simulink model "muscleLegs_task1"  (R2025b)
settings: Solver=ode23t  StartTime=0.0  StopTime=t_end  MaxStep=1e-3  RelTol=1e-4
values from neighbouring files (symbols this model uses):
  c = 0.05    [setup_muscleLegs_nm.m]
  CtrlPar = [tau_H_st; phi_K_tgt_st; P_K_st; D_K_st ... (first row only)    [setup_muscleLegs_ctrl.m]
  eref_se = 0.04    [setup_muscleLegs_nm.m]
  FmaxBFSH = 350    [setup_muscleLegs_nm.m]
  FmaxGLU = 4000    [setup_muscleLegs_nm.m]
  FmaxHFL = 2000    [setup_muscleLegs_nm.m]
  FmaxVAS = 5000    [setup_muscleLegs_nm.m]
  g = 9.81    [setup_muscleLegs_model.m]
  init_stim = 0.01    [setup_muscleLegs_nm.m]
  K = 5    [setup_muscleLegs_nm.m]
  l_shank = l_leg/2    (= 0.49)    [setup_muscleLegs_model.m]
  l_thigh = l_leg/2    (= 0.49)    [setup_muscleLegs_model.m]
  loptBFSH = 0.12    [setup_muscleLegs_nm.m]
  loptGLU = 0.11    [setup_muscleLegs_nm.m]
  loptHFL = 0.11    [setup_muscleLegs_nm.m]
  loptVAS = 0.08    [setup_muscleLegs_nm.m]
  lslackBFSH = 0.10    (= 0.1)    [setup_muscleLegs_nm.m]
  lslackGLU = 0.13    [setup_muscleLegs_nm.m]
  lslackHFL = 0.10    (= 0.1)    [setup_muscleLegs_nm.m]
  lslackVAS = 0.23    [setup_muscleLegs_nm.m]
  m_body = m_total - 2*m_foot    (= 78)    [setup_muscleLegs_model.m]
  m_shank = 4    [setup_muscleLegs_model.m]
  m_thigh = 8    [setup_muscleLegs_model.m]
  N = 12    [cmaes_task1_2_set1.mat]    (also in cmaes_task1_2_set2.mat; cmaes_task2_2_set1.mat = 17; cmaes_task2_2_set2.mat = 17; cmaes_task3_crouch.mat = 17)
  phirefBFSH = 160*pi/180    (= 2.79252680319)    [setup_muscleLegs_nm.m]
  phirefGLU = 60*pi/180    (= 1.0471975512)    [setup_muscleLegs_nm.m]
  phirefHFL = 20*pi/180    (= 0.349065850399)    [setup_muscleLegs_nm.m]
  phirefVAS = 60*pi/180    (= 1.0471975512)    [setup_muscleLegs_nm.m]
  plane_height = 0.1    [setup_muscleLegs_model.m]
  plane_x = 100    [setup_muscleLegs_model.m]
  plane_z = 1    [setup_muscleLegs_model.m]
  r_foot = 0.01    [setup_muscleLegs_model.m]
  rBFSH = 0.04    [setup_muscleLegs_nm.m]
  rGLU = 0.08    [setup_muscleLegs_nm.m]
  rHFL = 0.08    [setup_muscleLegs_nm.m]
  rhoBFSH = 0.7    [setup_muscleLegs_nm.m]
  rhoGLU = 0.5    [setup_muscleLegs_nm.m]
  rhoHFL = 0.5    [setup_muscleLegs_nm.m]
  rhoVAS = 0.6    [setup_muscleLegs_nm.m]
  rVAS = 0.05    [setup_muscleLegs_nm.m]
  tau_act = 0.01    [setup_muscleLegs_nm.m]
  tau_deact = 0.04    [setup_muscleLegs_nm.m]
  vi_Ctrl_st = 1:4    [setup_muscleLegs_ctrl.m]
  vi_Ctrl_sw = 5:12    [setup_muscleLegs_ctrl.m]
  vmaxBFSH = 12    [setup_muscleLegs_nm.m]
  vmaxGLU = 12    [setup_muscleLegs_nm.m]
  vmaxHFL = 12    [setup_muscleLegs_nm.m]
  vmaxVAS = 12    [setup_muscleLegs_nm.m]
  w = 0.56    [setup_muscleLegs_nm.m]
  w_pe = w    (= 0.56)    [setup_muscleLegs_nm.m]
undefined symbols (not defined in the file or in its folder): l1, X, Y, Z
libraries: sm_lib x30, nesl_utility x17, simulink x1
(part 2 of 4)

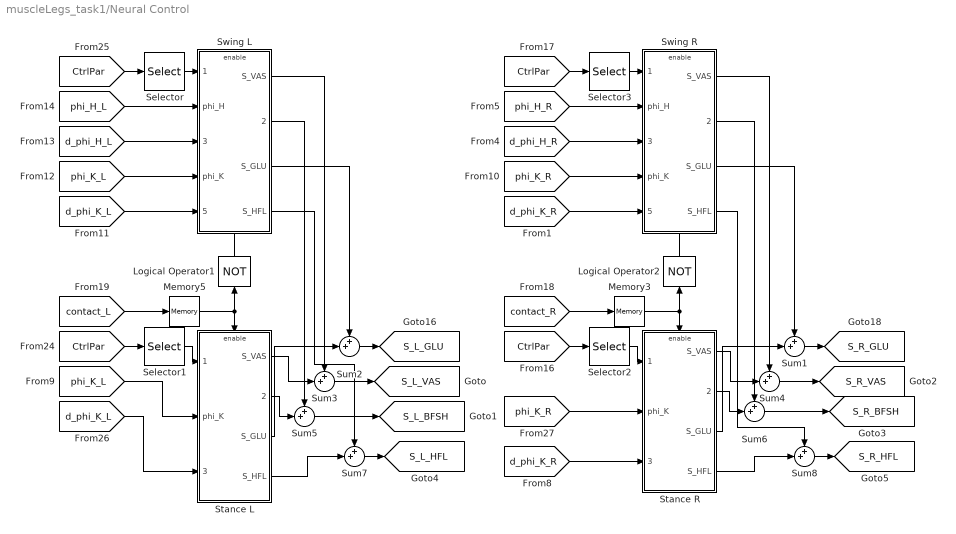
== system muscleLegs_task1/Neural Control ==
  Logical Operator1 : Logic  Operator=NOT  AllPortsSameDT=off  OutDataTypeStr=boolean
  Logical Operator2 : Logic  Operator=NOT  AllPortsSameDT=off  OutDataTypeStr=boolean
  Memory3 : Memory
  Memory5 : Memory  InitialCondition=1
  Selector : Selector  InputPortWidth=length(CtrlPar)  IndexOptions=Index vector (dialog)  Indices=vi_Ctrl_sw  OutputSizes=1
  Selector1 : Selector  InputPortWidth=length(CtrlPar)  IndexOptions=Index vector (dialog)  Indices=vi_Ctrl_st  OutputSizes=1
  Selector2 : Selector  InputPortWidth=length(CtrlPar)  IndexOptions=Index vector (dialog)  Indices=vi_Ctrl_st  OutputSizes=1
  Selector3 : Selector  InputPortWidth=length(CtrlPar)  IndexOptions=Index vector (dialog)  Indices=vi_Ctrl_sw  OutputSizes=1
  Stance L : Subsystem
  Stance R : Subsystem
  Sum{1..8} (8 alike) : Sum  Inputs=++|
  Swing L : Subsystem
  Swing R : Subsystem
  tag scope: S_L_BFSH=global, S_L_GLU=global, S_L_HFL=global, S_L_VAS=global, S_R_BFSH=global, S_R_GLU=global, S_R_HFL=global, S_R_VAS=global
  wires:
  [contact_R] -> Memory3/1
  [phi_K_R] -> Swing R/4(phi_K)
  Sum2/1 -> [S_L_GLU]
  Logical Operator1/1 -> Swing L/Enable
  Memory5/1 -> Logical Operator1/1, Stance L/Enable
  Selector1/1 -> Stance L/1(CtrlPar)
  [CtrlPar] -> Selector2/1
  Memory3/1 -> Stance R/Enable, Logical Operator2/1
  [phi_H_L] -> Swing L/2(phi_H)
  [d_phi_K_L] -> Stance L/3(d_phi_K)
  Logical Operator2/1 -> Swing R/Enable
  [d_phi_K_R] -> Stance R/3(d_phi_K)
  [d_phi_H_L] -> Swing L/3(d_phi_H)
  Sum1/1 -> [S_R_GLU]
  [d_phi_K_L] -> Swing L/5(d_phi_K)
  [d_phi_H_R] -> Swing R/3(d_phi_H)
  [d_phi_K_R] -> Swing R/5(d_phi_K)
  [phi_H_R] -> Swing R/2(phi_H)
  [CtrlPar] -> Selector/1
  [CtrlPar] -> Selector1/1
  Selector3/1 -> Swing R/1(CtrlPar)
  [phi_K_R] -> Stance R/2(phi_K)
  Selector/1 -> Swing L/1(CtrlPar)
  Selector2/1 -> Stance R/1(CtrlPar)
  [CtrlPar] -> Selector3/1
  [phi_K_L] -> Stance L/2(phi_K)
  [phi_K_L] -> Swing L/4(phi_K)
  [contact_L] -> Memory5/1
  Swing L/1(S_VAS) -> Sum3/1
  Swing L/2(S_BFSH) -> Sum5/1
  Sum3/1 -> [S_L_VAS]
  Stance L/1(S_VAS) -> Sum3/2
  Stance L/2(S_BFSH) -> Sum5/2
  Sum5/1 -> [S_L_BFSH]
  Stance R/2(S_BFSH) -> Sum6/2
  Stance R/1(S_VAS) -> Sum4/2
  Sum4/1 -> [S_R_VAS]
  Sum6/1 -> [S_R_BFSH]
  Swing R/2(S_BFSH) -> Sum6/1
  Swing R/1(S_VAS) -> Sum4/1
  Swing L/3(S_GLU) -> Sum2/1
  Stance L/3(S_GLU) -> Sum2/2
  Sum7/1 -> [S_L_HFL]
  Swing L/4(S_HFL) -> Sum7/1
  Stance L/4(S_HFL) -> Sum7/2
  Swing R/3(S_GLU) -> Sum1/1
  Stance R/3(S_GLU) -> Sum1/2
  Sum8/1 -> [S_R_HFL]
  Swing R/4(S_HFL) -> Sum8/1
  Stance R/4(S_HFL) -> Sum8/2

== system muscleLegs_task1/Muscle Dynamics/ECC ==
  S : Inport
  Constant : Constant  Value=tau_act
  Constant1 : Constant  Value=tau_deact
  Divide : Product  Inputs=*/
  Integrator : Integrator  InitialCondition=init_stim
  Sum : Sum  Inputs=+-|
  Switch : Switch  Criteria=u2 > Threshold  SaturateOnIntegerOverflow=off  InputSameDT=off
  Out1 : Outport
  A : Outport  Port=2  VectorParamsAs1DForOutWhenUnconnected=off
  wires:
  S/1 -> Sum/1
  Integrator/1 -> A/1, Sum/2  "A"
  Divide/1 -> Integrator/1  "dA"
  Sum/1 -> Divide/1, Switch/2
  Switch/1 -> Divide/2
  Constant/1 -> Switch/1
  Constant1/1 -> Switch/3

== system muscleLegs_task1/Muscle Dynamics/ECC1 ==
  S : Inport
  Constant : Constant  Value=tau_act
  Constant1 : Constant  Value=tau_deact
  Divide : Product  Inputs=*/
  Integrator : Integrator  InitialCondition=init_stim
  Sum : Sum  Inputs=+-|
  Switch : Switch  Criteria=u2 > Threshold  SaturateOnIntegerOverflow=off  InputSameDT=off
  A : Outport  VectorParamsAs1DForOutWhenUnconnected=off
  wires:
  S/1 -> Sum/1
  Integrator/1 -> A/1, Sum/2  "A"
  Divide/1 -> Integrator/1  "dA"
  Sum/1 -> Divide/1, Switch/2
  Switch/1 -> Divide/2
  Constant/1 -> Switch/1
  Constant1/1 -> Switch/3

== system muscleLegs_task1/Muscle Dynamics/ECC2 ==
  S : Inport
  Constant : Constant  Value=tau_act
  Constant1 : Constant  Value=tau_deact
  Divide : Product  Inputs=*/
  Integrator : Integrator  InitialCondition=init_stim
  Sum : Sum  Inputs=+-|
  Switch : Switch  Criteria=u2 > Threshold  SaturateOnIntegerOverflow=off  InputSameDT=off
  A : Outport  VectorParamsAs1DForOutWhenUnconnected=off
  wires:
  S/1 -> Sum/1
  Integrator/1 -> A/1, Sum/2  "A"
  Divide/1 -> Integrator/1  "dA"
  Sum/1 -> Divide/1, Switch/2
  Switch/1 -> Divide/2
  Constant/1 -> Switch/1
  Constant1/1 -> Switch/3

== system muscleLegs_task1/Muscle Dynamics/ECC3 ==
  S : Inport
  Constant : Constant  Value=tau_act
  Constant1 : Constant  Value=tau_deact
  Divide : Product  Inputs=*/
  Integrator : Integrator  InitialCondition=init_stim
  Sum : Sum  Inputs=+-|
  Switch : Switch  Criteria=u2 > Threshold  SaturateOnIntegerOverflow=off  InputSameDT=off
  A : Outport  VectorParamsAs1DForOutWhenUnconnected=off
  wires:
  S/1 -> Sum/1
  Integrator/1 -> A/1, Sum/2  "A"
  Divide/1 -> Integrator/1  "dA"
  Sum/1 -> Divide/1, Switch/2
  Switch/1 -> Divide/2
  Constant/1 -> Switch/1
  Constant1/1 -> Switch/3

== system muscleLegs_task1/Muscle Dynamics/ECC4 ==
  S : Inport
  Constant : Constant  Value=tau_act
  Constant1 : Constant  Value=tau_deact
  Divide : Product  Inputs=*/
  Integrator : Integrator  InitialCondition=init_stim
  Sum : Sum  Inputs=+-|
  Switch : Switch  Criteria=u2 > Threshold  SaturateOnIntegerOverflow=off  InputSameDT=off
  A : Outport  VectorParamsAs1DForOutWhenUnconnected=off
  wires:
  S/1 -> Sum/1
  Integrator/1 -> A/1, Sum/2  "A"
  Divide/1 -> Integrator/1  "dA"
  Sum/1 -> Divide/1, Switch/2
  Switch/1 -> Divide/2
  Constant/1 -> Switch/1
  Constant1/1 -> Switch/3

== system muscleLegs_task1/Muscle Dynamics/ECC5 ==
  S : Inport
  Constant : Constant  Value=tau_act
  Constant1 : Constant  Value=tau_deact
  Divide : Product  Inputs=*/
  Integrator : Integrator  InitialCondition=init_stim
  Sum : Sum  Inputs=+-|
  Switch : Switch  Criteria=u2 > Threshold  SaturateOnIntegerOverflow=off  InputSameDT=off
  A : Outport  VectorParamsAs1DForOutWhenUnconnected=off
  wires:
  S/1 -> Sum/1
  Integrator/1 -> A/1, Sum/2  "A"
  Divide/1 -> Integrator/1  "dA"
  Sum/1 -> Divide/1, Switch/2
  Switch/1 -> Divide/2
  Constant/1 -> Switch/1
  Constant1/1 -> Switch/3

== system muscleLegs_task1/Muscle Dynamics/ECC6 ==
  S : Inport
  Constant : Constant  Value=tau_act
  Constant1 : Constant  Value=tau_deact
  Divide : Product  Inputs=*/
  Integrator : Integrator  InitialCondition=init_stim
  Sum : Sum  Inputs=+-|
  Switch : Switch  Criteria=u2 > Threshold  SaturateOnIntegerOverflow=off  InputSameDT=off
  A : Outport  VectorParamsAs1DForOutWhenUnconnected=off
  wires:
  S/1 -> Sum/1
  Integrator/1 -> A/1, Sum/2  "A"
  Divide/1 -> Integrator/1  "dA"
  Sum/1 -> Divide/1, Switch/2
  Switch/1 -> Divide/2
  Constant/1 -> Switch/1
  Constant1/1 -> Switch/3

== system muscleLegs_task1/Muscle Dynamics/ECC7 ==
  S : Inport
  Constant : Constant  Value=tau_act
  Constant1 : Constant  Value=tau_deact
  Divide : Product  Inputs=*/
  Integrator : Integrator  InitialCondition=init_stim
  Sum : Sum  Inputs=+-|
  Switch : Switch  Criteria=u2 > Threshold  SaturateOnIntegerOverflow=off  InputSameDT=off
  A : Outport  VectorParamsAs1DForOutWhenUnconnected=off
  wires:
  S/1 -> Sum/1
  Integrator/1 -> A/1, Sum/2  "A"
  Divide/1 -> Integrator/1  "dA"
  Sum/1 -> Divide/1, Switch/2
  Switch/1 -> Divide/2
  Constant/1 -> Switch/1
  Constant1/1 -> Switch/3

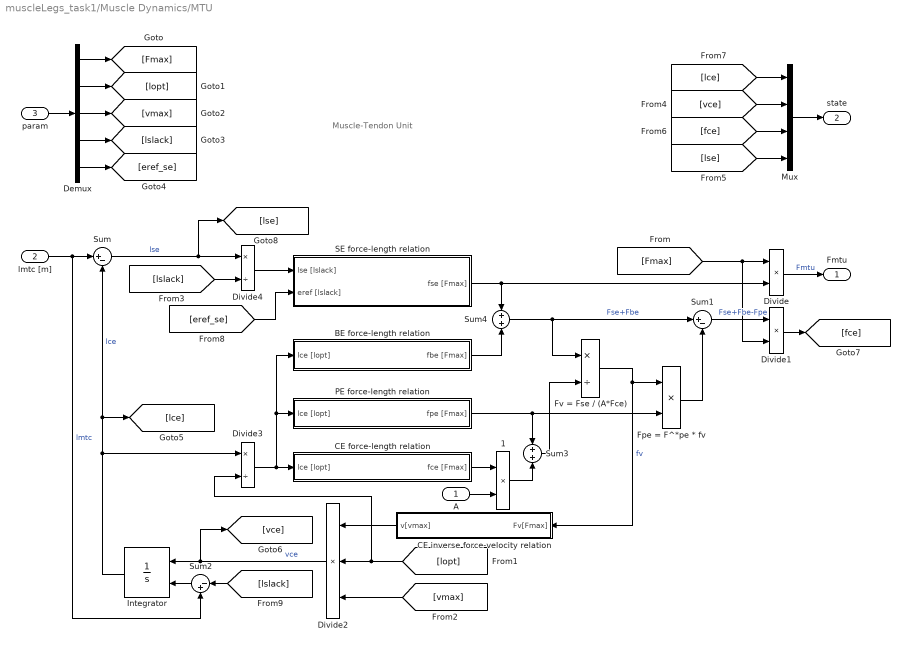
== system muscleLegs_task1/Muscle Dynamics/MTU ==
  note: Muscle-Tendon Unit
  A : Inport
  lmtc [m] : Inport  Port=2
  param : Inport  Port=3
  1 : Product  Inputs=**  InputSameDT=on  SaturateOnIntegerOverflow=on  OutDataTypeStr=Inherit: Same as first input
  BE force-length relation : Subsystem
  CE force-length relation : Subsystem
  CE inverse force-velocity relation : Subsystem
  Demux : Demux  Outputs=5
  Divide : Product
  Divide1 : Product
  Divide2 : Product  Inputs=3
  Divide3 : Product  Inputs=*/
  Divide4 : Product  Inputs=*/
  "Fpe = F^*pe * fv " : Product  InputSameDT=on  SaturateOnIntegerOverflow=on  OutDataTypeStr=Inherit: Same as first input
  Fv = Fse / (A*Fce) : Product  Inputs=*/  InputSameDT=on  SaturateOnIntegerOverflow=on  OutDataTypeStr=Inherit: Same as first input
  Integrator : Integrator  InitialConditionSource=external  LowerSaturationLimit=0.05
  Mux : Mux
  PE force-length relation : Subsystem
  SE force-length relation : Subsystem
  Sum : Sum  Inputs=|+-  InputSameDT=on  SaturateOnIntegerOverflow=on  OutDataTypeStr=Inherit: Same as first input
  Sum1 : Sum  Inputs=|+-  InputSameDT=on  SaturateOnIntegerOverflow=on  OutDataTypeStr=Inherit: Same as first input
  Sum2 : Sum  Inputs=|-+  InputSameDT=on  SaturateOnIntegerOverflow=on  OutDataTypeStr=Inherit: Same as first input
  Sum3 : Sum  InputSameDT=on  SaturateOnIntegerOverflow=on  OutDataTypeStr=Inherit: Same as first input
  Sum4 : Sum  InputSameDT=on  SaturateOnIntegerOverflow=on  OutDataTypeStr=Inherit: Same as first input
  Fmtu : Outport  InitialOutput=0  VectorParamsAs1DForOutWhenUnconnected=off
  state : Outport  Port=2  InitialOutput=0  VectorParamsAs1DForOutWhenUnconnected=off
  wires:
  Integrator/1 -> Divide3/1, [lce], Sum/2  "lce"
  Divide3/1 -> CE force-length relation/1(lce [lopt]), PE force-length relation/1(lce [lopt]), BE force-length relation/1(lce [lopt])
  Fv = Fse / (A*Fce)/1 -> CE inverse force-velocity relation/1(Fv[Fmax]), "Fpe = F^*pe * fv "/1  "fv"
  Divide2/1 -> [vce], Integrator/1  "vce"
  lmtc [m]/1 -> Sum/1, Sum2/2  "lmtc"
  Divide/1 -> Fmtu/1  "Fmtu"
  Divide4/1 -> SE force-length relation/1(lse [lslack])
  SE force-length relation/1(fse [Fmax]) -> Sum4/1, Divide/2
  Sum2/1 -> Integrator/2
  [lslack] -> Sum2/1
  CE force-length relation/1(fce [Fmax]) -> 1/1
  PE force-length relation/1(fpe [Fmax]) -> "Fpe = F^*pe * fv "/2, Sum3/1
  1/1 -> Sum3/2
  BE force-length relation/1(fbe [Fmax]) -> Sum4/2
  Sum3/1 -> Fv = Fse / (A*Fce)/2
  CE inverse force-velocity relation/1(v[vmax]) -> Divide2/1
  A/1 -> 1/2
  Sum4/1 -> Sum1/1, Fv = Fse / (A*Fce)/1  "Fse+Fbe"
  "Fpe = F^*pe * fv "/1 -> Sum1/2
  Sum1/1 -> Divide1/1  "Fse+Fbe-Fpe"
  Divide1/1 -> [fce]
  Sum/1 -> [lse], Divide4/1  "lse"
  [lopt] -> Divide2/2, Divide3/2
  [vmax] -> Divide2/3
  [lslack] -> Divide4/2
  param/1 -> Demux/1
  Demux/1 -> [Fmax]
  Demux/2 -> [lopt]
  Demux/4 -> [lslack]
  Demux/3 -> [vmax]
  Demux/5 -> [eref_se]
  [Fmax] -> Divide1/2, Divide/1
  Mux/1 -> state/1
  [lce] -> Mux/1
  [vce] -> Mux/2
  [fce] -> Mux/3
  [lse] -> Mux/4
  [eref_se] -> SE force-length relation/2(eref [lslack])

== system muscleLegs_task1/Muscle Dynamics/MTU Link ==
  note: check sign:
      | ++: larger phi -> longer mtu
      | +-: larger phi -> shorter mtu
  note: Muscle Attachment
  phi [rad] : Inport
  param : Inport  Port=2
  Demux : Demux  Outputs=5
  Product : Product  Inputs=3  RndMeth=Zero
  Sum1 : Sum  Inputs=|++
  Sum2 : Sum  Inputs=|+-
  Sum5 : Sum  Inputs=|++
  lmtu [m] : Outport  VectorParamsAs1DForOutWhenUnconnected=off
  lever [m] : Outport  Port=2  VectorParamsAs1DForOutWhenUnconnected=off
  wires:
  Sum1/1 -> Sum5/1
  Sum5/1 -> lmtu [m]/1
  phi [rad]/1 -> Sum2/1
  Demux/3 -> Sum2/2  "phiref"
  Sum2/1 -> Product/1
  Demux/4 -> lever [m]/1, Product/2  "r"
  Product/1 -> Sum5/2
  Demux/1 -> Sum1/1  "lopt"
  Demux/2 -> Sum1/2  "lslack"
  Demux/5 -> Product/3  "rho"
  param/1 -> Demux/1

== system muscleLegs_task1/Muscle Dynamics/MTU Link1 ==
  note: check sign:
      | ++: larger phi -> longer mtu
      | +-: larger phi -> shorter mtu
  note: Muscle Attachment
  phi [rad] : Inport
  param : Inport  Port=2
  Demux : Demux  Outputs=5
  Product : Product  Inputs=3  RndMeth=Zero
  Sum1 : Sum  Inputs=|++
  Sum2 : Sum  Inputs=|+-
  Sum5 : Sum  Inputs=|+-
  lmtu [m] : Outport  VectorParamsAs1DForOutWhenUnconnected=off
  lever [m] : Outport  Port=2  VectorParamsAs1DForOutWhenUnconnected=off
  wires:
  Sum1/1 -> Sum5/1
  Sum5/1 -> lmtu [m]/1
  phi [rad]/1 -> Sum2/1
  Demux/3 -> Sum2/2  "phiref"
  Sum2/1 -> Product/1
  Demux/4 -> lever [m]/1, Product/2  "r"
  Product/1 -> Sum5/2
  Demux/1 -> Sum1/1  "lopt"
  Demux/2 -> Sum1/2  "lslack"
  Demux/5 -> Product/3  "rho"
  param/1 -> Demux/1

== system muscleLegs_task1/Muscle Dynamics/MTU Link2 ==
  note: check sign:
      | ++: larger phi -> longer mtu
      | +-: larger phi -> shorter mtu
  note: Muscle Attachment
  phi [rad] : Inport
  param : Inport  Port=2
  Demux : Demux  Outputs=5
  Product : Product  Inputs=3  RndMeth=Zero
  Sum1 : Sum  Inputs=|++
  Sum2 : Sum  Inputs=|+-
  Sum5 : Sum  Inputs=|++
  lmtu [m] : Outport  VectorParamsAs1DForOutWhenUnconnected=off
  lever [m] : Outport  Port=2  VectorParamsAs1DForOutWhenUnconnected=off
  wires:
  Sum1/1 -> Sum5/1
  Sum5/1 -> lmtu [m]/1
  phi [rad]/1 -> Sum2/1
  Demux/3 -> Sum2/2  "phiref"
  Sum2/1 -> Product/1
  Demux/4 -> lever [m]/1, Product/2  "r"
  Product/1 -> Sum5/2
  Demux/1 -> Sum1/1  "lopt"
  Demux/2 -> Sum1/2  "lslack"
  Demux/5 -> Product/3  "rho"
  param/1 -> Demux/1

== system muscleLegs_task1/Muscle Dynamics/MTU Link3 ==
  note: check sign:
      | ++: larger phi -> longer mtu
      | +-: larger phi -> shorter mtu
  note: Muscle Attachment
  phi [rad] : Inport
  param : Inport  Port=2
  Demux : Demux  Outputs=5
  Product : Product  Inputs=3  RndMeth=Zero
  Sum1 : Sum  Inputs=|++
  Sum2 : Sum  Inputs=|+-
  Sum5 : Sum  Inputs=|+-
  lmtu [m] : Outport  VectorParamsAs1DForOutWhenUnconnected=off
  lever [m] : Outport  Port=2  VectorParamsAs1DForOutWhenUnconnected=off
  wires:
  Sum1/1 -> Sum5/1
  Sum5/1 -> lmtu [m]/1
  phi [rad]/1 -> Sum2/1
  Demux/3 -> Sum2/2  "phiref"
  Sum2/1 -> Product/1
  Demux/4 -> lever [m]/1, Product/2  "r"
  Product/1 -> Sum5/2
  Demux/1 -> Sum1/1  "lopt"
  Demux/2 -> Sum1/2  "lslack"
  Demux/5 -> Product/3  "rho"
  param/1 -> Demux/1

== system muscleLegs_task1/Muscle Dynamics/MTU Link4 ==
  note: check sign:
      | ++: larger phi -> longer mtu
      | +-: larger phi -> shorter mtu
  note: Muscle Attachment
  phi [rad] : Inport
  param : Inport  Port=2
  Demux : Demux  Outputs=5
  Product : Product  Inputs=3  RndMeth=Zero
  Sum1 : Sum  Inputs=|++
  Sum2 : Sum  Inputs=|+-
  Sum5 : Sum  Inputs=|++
  lmtu [m] : Outport  VectorParamsAs1DForOutWhenUnconnected=off
  lever [m] : Outport  Port=2  VectorParamsAs1DForOutWhenUnconnected=off
  wires:
  Sum1/1 -> Sum5/1
  Sum5/1 -> lmtu [m]/1
  phi [rad]/1 -> Sum2/1
  Demux/3 -> Sum2/2  "phiref"
  Sum2/1 -> Product/1
  Demux/4 -> lever [m]/1, Product/2  "r"
  Product/1 -> Sum5/2
  Demux/1 -> Sum1/1  "lopt"
  Demux/2 -> Sum1/2  "lslack"
  Demux/5 -> Product/3  "rho"
  param/1 -> Demux/1

== system muscleLegs_task1/Muscle Dynamics/MTU Link5 ==
  note: check sign:
      | ++: larger phi -> longer mtu
      | +-: larger phi -> shorter mtu
  note: Muscle Attachment
  phi [rad] : Inport
  param : Inport  Port=2
  Demux : Demux  Outputs=5
  Product : Product  Inputs=3  RndMeth=Zero
  Sum1 : Sum  Inputs=|++
  Sum2 : Sum  Inputs=|+-
  Sum5 : Sum  Inputs=|+-
  lmtu [m] : Outport  VectorParamsAs1DForOutWhenUnconnected=off
  lever [m] : Outport  Port=2  VectorParamsAs1DForOutWhenUnconnected=off
  wires:
  Sum1/1 -> Sum5/1
  Sum5/1 -> lmtu [m]/1
  phi [rad]/1 -> Sum2/1
  Demux/3 -> Sum2/2  "phiref"
  Sum2/1 -> Product/1
  Demux/4 -> lever [m]/1, Product/2  "r"
  Product/1 -> Sum5/2
  Demux/1 -> Sum1/1  "lopt"
  Demux/2 -> Sum1/2  "lslack"
  Demux/5 -> Product/3  "rho"
  param/1 -> Demux/1

== system muscleLegs_task1/Muscle Dynamics/MTU Link6 ==
  note: check sign:
      | ++: larger phi -> longer mtu
      | +-: larger phi -> shorter mtu
  note: Muscle Attachment
  phi [rad] : Inport
  param : Inport  Port=2
  Demux : Demux  Outputs=5
  Product : Product  Inputs=3  RndMeth=Zero
  Sum1 : Sum  Inputs=|++
  Sum2 : Sum  Inputs=|+-
  Sum5 : Sum  Inputs=|++
  lmtu [m] : Outport  VectorParamsAs1DForOutWhenUnconnected=off
  lever [m] : Outport  Port=2  VectorParamsAs1DForOutWhenUnconnected=off
  wires:
  Sum1/1 -> Sum5/1
  Sum5/1 -> lmtu [m]/1
  phi [rad]/1 -> Sum2/1
  Demux/3 -> Sum2/2  "phiref"
  Sum2/1 -> Product/1
  Demux/4 -> lever [m]/1, Product/2  "r"
  Product/1 -> Sum5/2
  Demux/1 -> Sum1/1  "lopt"
  Demux/2 -> Sum1/2  "lslack"
  Demux/5 -> Product/3  "rho"
  param/1 -> Demux/1

== system muscleLegs_task1/Muscle Dynamics/MTU Link7 ==
  note: check sign:
      | ++: larger phi -> longer mtu
      | +-: larger phi -> shorter mtu
  note: Muscle Attachment
  phi [rad] : Inport
  param : Inport  Port=2
  Demux : Demux  Outputs=5
  Product : Product  Inputs=3  RndMeth=Zero
  Sum1 : Sum  Inputs=|++
  Sum2 : Sum  Inputs=|+-
  Sum5 : Sum  Inputs=|+-
  lmtu [m] : Outport  VectorParamsAs1DForOutWhenUnconnected=off
  lever [m] : Outport  Port=2  VectorParamsAs1DForOutWhenUnconnected=off
  wires:
  Sum1/1 -> Sum5/1
  Sum5/1 -> lmtu [m]/1
  phi [rad]/1 -> Sum2/1
  Demux/3 -> Sum2/2  "phiref"
  Sum2/1 -> Product/1
  Demux/4 -> lever [m]/1, Product/2  "r"
  Product/1 -> Sum5/2
  Demux/1 -> Sum1/1  "lopt"
  Demux/2 -> Sum1/2  "lslack"
  Demux/5 -> Product/3  "rho"
  param/1 -> Demux/1

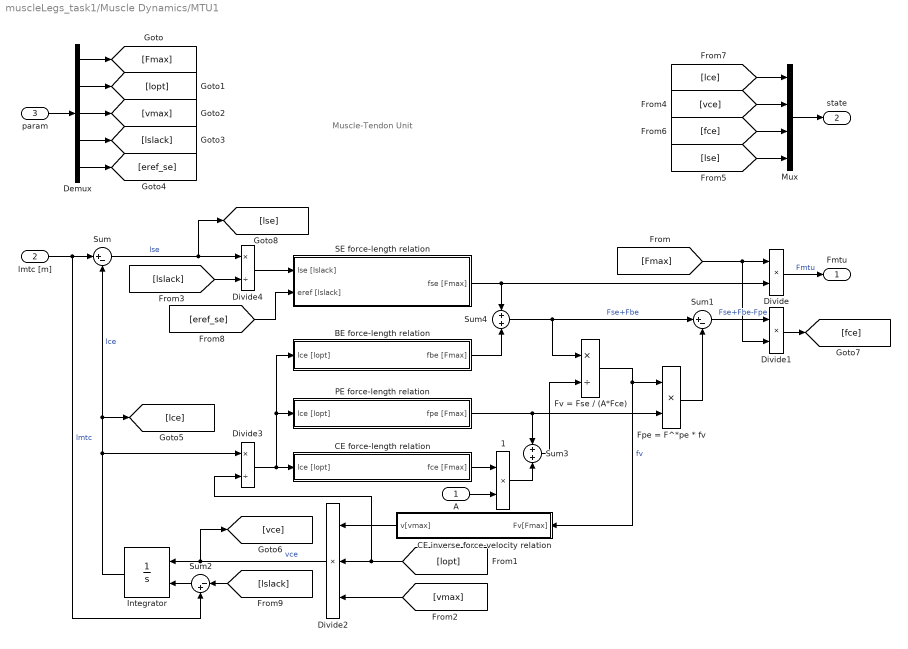
== system muscleLegs_task1/Muscle Dynamics/MTU1 ==
  note: Muscle-Tendon Unit
  A : Inport
  lmtc [m] : Inport  Port=2
  param : Inport  Port=3
  1 : Product  Inputs=**  InputSameDT=on  SaturateOnIntegerOverflow=on  OutDataTypeStr=Inherit: Same as first input
  BE force-length relation : Subsystem
  CE force-length relation : Subsystem
  CE inverse force-velocity relation : Subsystem
  Demux : Demux  Outputs=5
  Divide : Product
  Divide1 : Product
  Divide2 : Product  Inputs=3
  Divide3 : Product  Inputs=*/
  Divide4 : Product  Inputs=*/
  "Fpe = F^*pe * fv " : Product  InputSameDT=on  SaturateOnIntegerOverflow=on  OutDataTypeStr=Inherit: Same as first input
  Fv = Fse / (A*Fce) : Product  Inputs=*/  InputSameDT=on  SaturateOnIntegerOverflow=on  OutDataTypeStr=Inherit: Same as first input
  Integrator : Integrator  InitialConditionSource=external  LowerSaturationLimit=0.05
  Mux : Mux
  PE force-length relation : Subsystem
  SE force-length relation : Subsystem
  Sum : Sum  Inputs=|+-  InputSameDT=on  SaturateOnIntegerOverflow=on  OutDataTypeStr=Inherit: Same as first input
  Sum1 : Sum  Inputs=|+-  InputSameDT=on  SaturateOnIntegerOverflow=on  OutDataTypeStr=Inherit: Same as first input
  Sum2 : Sum  Inputs=|-+  InputSameDT=on  SaturateOnIntegerOverflow=on  OutDataTypeStr=Inherit: Same as first input
  Sum3 : Sum  InputSameDT=on  SaturateOnIntegerOverflow=on  OutDataTypeStr=Inherit: Same as first input
  Sum4 : Sum  InputSameDT=on  SaturateOnIntegerOverflow=on  OutDataTypeStr=Inherit: Same as first input
  Fmtu : Outport  InitialOutput=0  VectorParamsAs1DForOutWhenUnconnected=off
  state : Outport  Port=2  InitialOutput=0  VectorParamsAs1DForOutWhenUnconnected=off
  wires:
  Integrator/1 -> Divide3/1, [lce], Sum/2  "lce"
  Divide3/1 -> CE force-length relation/1(lce [lopt]), PE force-length relation/1(lce [lopt]), BE force-length relation/1(lce [lopt])
  Fv = Fse / (A*Fce)/1 -> CE inverse force-velocity relation/1(Fv[Fmax]), "Fpe = F^*pe * fv "/1  "fv"
  Divide2/1 -> [vce], Integrator/1  "vce"
  lmtc [m]/1 -> Sum/1, Sum2/2  "lmtc"
  Divide/1 -> Fmtu/1  "Fmtu"
  Divide4/1 -> SE force-length relation/1(lse [lslack])
  SE force-length relation/1(fse [Fmax]) -> Sum4/1, Divide/2
  Sum2/1 -> Integrator/2
  [lslack] -> Sum2/1
  CE force-length relation/1(fce [Fmax]) -> 1/1
  PE force-length relation/1(fpe [Fmax]) -> "Fpe = F^*pe * fv "/2, Sum3/1
  1/1 -> Sum3/2
  BE force-length relation/1(fbe [Fmax]) -> Sum4/2
  Sum3/1 -> Fv = Fse / (A*Fce)/2
  CE inverse force-velocity relation/1(v[vmax]) -> Divide2/1
  A/1 -> 1/2
  Sum4/1 -> Sum1/1, Fv = Fse / (A*Fce)/1  "Fse+Fbe"
  "Fpe = F^*pe * fv "/1 -> Sum1/2
  Sum1/1 -> Divide1/1  "Fse+Fbe-Fpe"
  Divide1/1 -> [fce]
  Sum/1 -> [lse], Divide4/1  "lse"
  [lopt] -> Divide2/2, Divide3/2
  [vmax] -> Divide2/3
  [lslack] -> Divide4/2
  param/1 -> Demux/1
  Demux/1 -> [Fmax]
  Demux/2 -> [lopt]
  Demux/4 -> [lslack]
  Demux/3 -> [vmax]
  Demux/5 -> [eref_se]
  [Fmax] -> Divide1/2, Divide/1
  Mux/1 -> state/1
  [lce] -> Mux/1
  [vce] -> Mux/2
  [fce] -> Mux/3
  [lse] -> Mux/4
  [eref_se] -> SE force-length relation/2(eref [lslack])

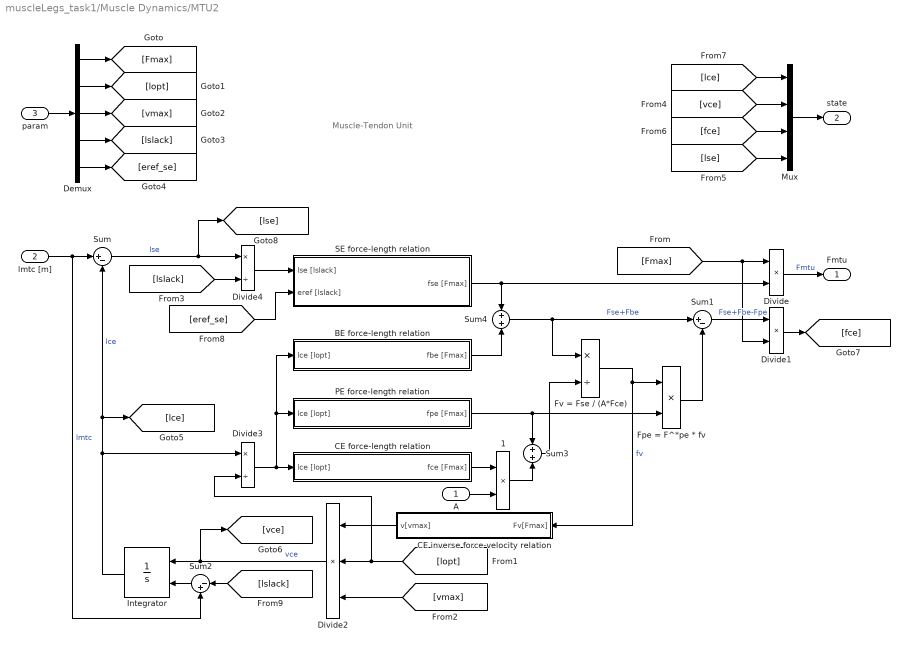
== system muscleLegs_task1/Muscle Dynamics/MTU2 ==
  note: Muscle-Tendon Unit
  A : Inport
  lmtc [m] : Inport  Port=2
  param : Inport  Port=3
  1 : Product  Inputs=**  InputSameDT=on  SaturateOnIntegerOverflow=on  OutDataTypeStr=Inherit: Same as first input
  BE force-length relation : Subsystem
  CE force-length relation : Subsystem
  CE inverse force-velocity relation : Subsystem
  Demux : Demux  Outputs=5
  Divide : Product
  Divide1 : Product
  Divide2 : Product  Inputs=3
  Divide3 : Product  Inputs=*/
  Divide4 : Product  Inputs=*/
  "Fpe = F^*pe * fv " : Product  InputSameDT=on  SaturateOnIntegerOverflow=on  OutDataTypeStr=Inherit: Same as first input
  Fv = Fse / (A*Fce) : Product  Inputs=*/  InputSameDT=on  SaturateOnIntegerOverflow=on  OutDataTypeStr=Inherit: Same as first input
  Integrator : Integrator  InitialConditionSource=external  LowerSaturationLimit=0.05
  Mux : Mux
  PE force-length relation : Subsystem
  SE force-length relation : Subsystem
  Sum : Sum  Inputs=|+-  InputSameDT=on  SaturateOnIntegerOverflow=on  OutDataTypeStr=Inherit: Same as first input
  Sum1 : Sum  Inputs=|+-  InputSameDT=on  SaturateOnIntegerOverflow=on  OutDataTypeStr=Inherit: Same as first input
  Sum2 : Sum  Inputs=|-+  InputSameDT=on  SaturateOnIntegerOverflow=on  OutDataTypeStr=Inherit: Same as first input
  Sum3 : Sum  InputSameDT=on  SaturateOnIntegerOverflow=on  OutDataTypeStr=Inherit: Same as first input
  Sum4 : Sum  InputSameDT=on  SaturateOnIntegerOverflow=on  OutDataTypeStr=Inherit: Same as first input
  Fmtu : Outport  InitialOutput=0  VectorParamsAs1DForOutWhenUnconnected=off
  state : Outport  Port=2  InitialOutput=0  VectorParamsAs1DForOutWhenUnconnected=off
  wires:
  Integrator/1 -> Divide3/1, [lce], Sum/2  "lce"
  Divide3/1 -> CE force-length relation/1(lce [lopt]), PE force-length relation/1(lce [lopt]), BE force-length relation/1(lce [lopt])
  Fv = Fse / (A*Fce)/1 -> CE inverse force-velocity relation/1(Fv[Fmax]), "Fpe = F^*pe * fv "/1  "fv"
  Divide2/1 -> [vce], Integrator/1  "vce"
  lmtc [m]/1 -> Sum/1, Sum2/2  "lmtc"
  Divide/1 -> Fmtu/1  "Fmtu"
  Divide4/1 -> SE force-length relation/1(lse [lslack])
  SE force-length relation/1(fse [Fmax]) -> Sum4/1, Divide/2
  Sum2/1 -> Integrator/2
  [lslack] -> Sum2/1
  CE force-length relation/1(fce [Fmax]) -> 1/1
  PE force-length relation/1(fpe [Fmax]) -> "Fpe = F^*pe * fv "/2, Sum3/1
  1/1 -> Sum3/2
  BE force-length relation/1(fbe [Fmax]) -> Sum4/2
  Sum3/1 -> Fv = Fse / (A*Fce)/2
  CE inverse force-velocity relation/1(v[vmax]) -> Divide2/1
  A/1 -> 1/2
  Sum4/1 -> Sum1/1, Fv = Fse / (A*Fce)/1  "Fse+Fbe"
  "Fpe = F^*pe * fv "/1 -> Sum1/2
  Sum1/1 -> Divide1/1  "Fse+Fbe-Fpe"
  Divide1/1 -> [fce]
  Sum/1 -> [lse], Divide4/1  "lse"
  [lopt] -> Divide2/2, Divide3/2
  [vmax] -> Divide2/3
  [lslack] -> Divide4/2
  param/1 -> Demux/1
  Demux/1 -> [Fmax]
  Demux/2 -> [lopt]
  Demux/4 -> [lslack]
  Demux/3 -> [vmax]
  Demux/5 -> [eref_se]
  [Fmax] -> Divide1/2, Divide/1
  Mux/1 -> state/1
  [lce] -> Mux/1
  [vce] -> Mux/2
  [fce] -> Mux/3
  [lse] -> Mux/4
  [eref_se] -> SE force-length relation/2(eref [lslack])

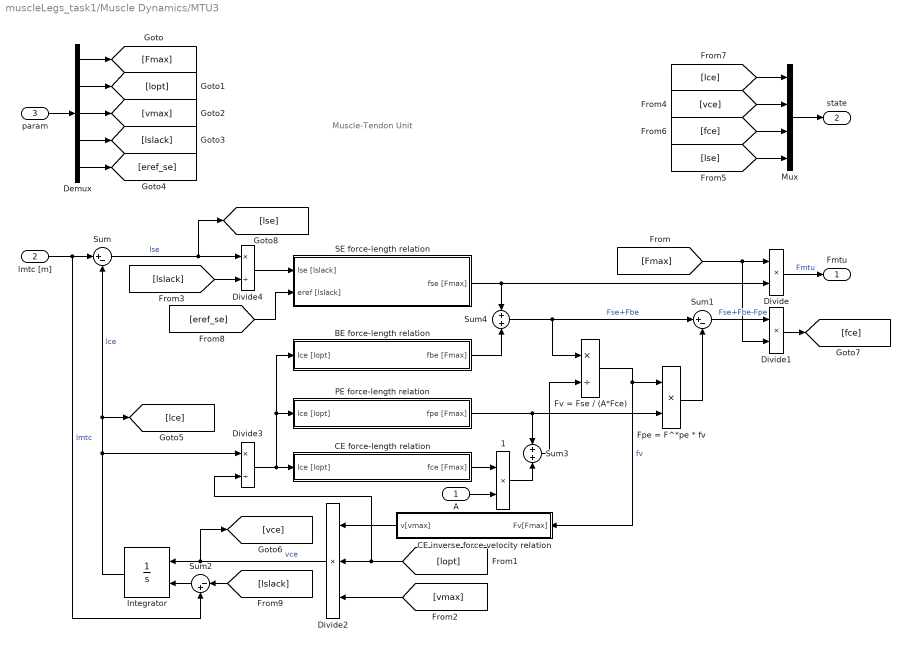
== system muscleLegs_task1/Muscle Dynamics/MTU3 ==
  note: Muscle-Tendon Unit
  A : Inport
  lmtc [m] : Inport  Port=2
  param : Inport  Port=3
  1 : Product  Inputs=**  InputSameDT=on  SaturateOnIntegerOverflow=on  OutDataTypeStr=Inherit: Same as first input
  BE force-length relation : Subsystem
  CE force-length relation : Subsystem
  CE inverse force-velocity relation : Subsystem
  Demux : Demux  Outputs=5
  Divide : Product
  Divide1 : Product
  Divide2 : Product  Inputs=3
  Divide3 : Product  Inputs=*/
  Divide4 : Product  Inputs=*/
  "Fpe = F^*pe * fv " : Product  InputSameDT=on  SaturateOnIntegerOverflow=on  OutDataTypeStr=Inherit: Same as first input
  Fv = Fse / (A*Fce) : Product  Inputs=*/  InputSameDT=on  SaturateOnIntegerOverflow=on  OutDataTypeStr=Inherit: Same as first input
  Integrator : Integrator  InitialConditionSource=external  LowerSaturationLimit=0.05
  Mux : Mux
  PE force-length relation : Subsystem
  SE force-length relation : Subsystem
  Sum : Sum  Inputs=|+-  InputSameDT=on  SaturateOnIntegerOverflow=on  OutDataTypeStr=Inherit: Same as first input
  Sum1 : Sum  Inputs=|+-  InputSameDT=on  SaturateOnIntegerOverflow=on  OutDataTypeStr=Inherit: Same as first input
  Sum2 : Sum  Inputs=|-+  InputSameDT=on  SaturateOnIntegerOverflow=on  OutDataTypeStr=Inherit: Same as first input
  Sum3 : Sum  InputSameDT=on  SaturateOnIntegerOverflow=on  OutDataTypeStr=Inherit: Same as first input
  Sum4 : Sum  InputSameDT=on  SaturateOnIntegerOverflow=on  OutDataTypeStr=Inherit: Same as first input
  Fmtu : Outport  InitialOutput=0  VectorParamsAs1DForOutWhenUnconnected=off
  state : Outport  Port=2  InitialOutput=0  VectorParamsAs1DForOutWhenUnconnected=off
  wires:
  Integrator/1 -> Divide3/1, [lce], Sum/2  "lce"
  Divide3/1 -> CE force-length relation/1(lce [lopt]), PE force-length relation/1(lce [lopt]), BE force-length relation/1(lce [lopt])
  Fv = Fse / (A*Fce)/1 -> CE inverse force-velocity relation/1(Fv[Fmax]), "Fpe = F^*pe * fv "/1  "fv"
  Divide2/1 -> [vce], Integrator/1  "vce"
  lmtc [m]/1 -> Sum/1, Sum2/2  "lmtc"
  Divide/1 -> Fmtu/1  "Fmtu"
  Divide4/1 -> SE force-length relation/1(lse [lslack])
  SE force-length relation/1(fse [Fmax]) -> Sum4/1, Divide/2
  Sum2/1 -> Integrator/2
  [lslack] -> Sum2/1
  CE force-length relation/1(fce [Fmax]) -> 1/1
  PE force-length relation/1(fpe [Fmax]) -> "Fpe = F^*pe * fv "/2, Sum3/1
  1/1 -> Sum3/2
  BE force-length relation/1(fbe [Fmax]) -> Sum4/2
  Sum3/1 -> Fv = Fse / (A*Fce)/2
  CE inverse force-velocity relation/1(v[vmax]) -> Divide2/1
  A/1 -> 1/2
  Sum4/1 -> Sum1/1, Fv = Fse / (A*Fce)/1  "Fse+Fbe"
  "Fpe = F^*pe * fv "/1 -> Sum1/2
  Sum1/1 -> Divide1/1  "Fse+Fbe-Fpe"
  Divide1/1 -> [fce]
  Sum/1 -> [lse], Divide4/1  "lse"
  [lopt] -> Divide2/2, Divide3/2
  [vmax] -> Divide2/3
  [lslack] -> Divide4/2
  param/1 -> Demux/1
  Demux/1 -> [Fmax]
  Demux/2 -> [lopt]
  Demux/4 -> [lslack]
  Demux/3 -> [vmax]
  Demux/5 -> [eref_se]
  [Fmax] -> Divide1/2, Divide/1
  Mux/1 -> state/1
  [lce] -> Mux/1
  [vce] -> Mux/2
  [fce] -> Mux/3
  [lse] -> Mux/4
  [eref_se] -> SE force-length relation/2(eref [lslack])

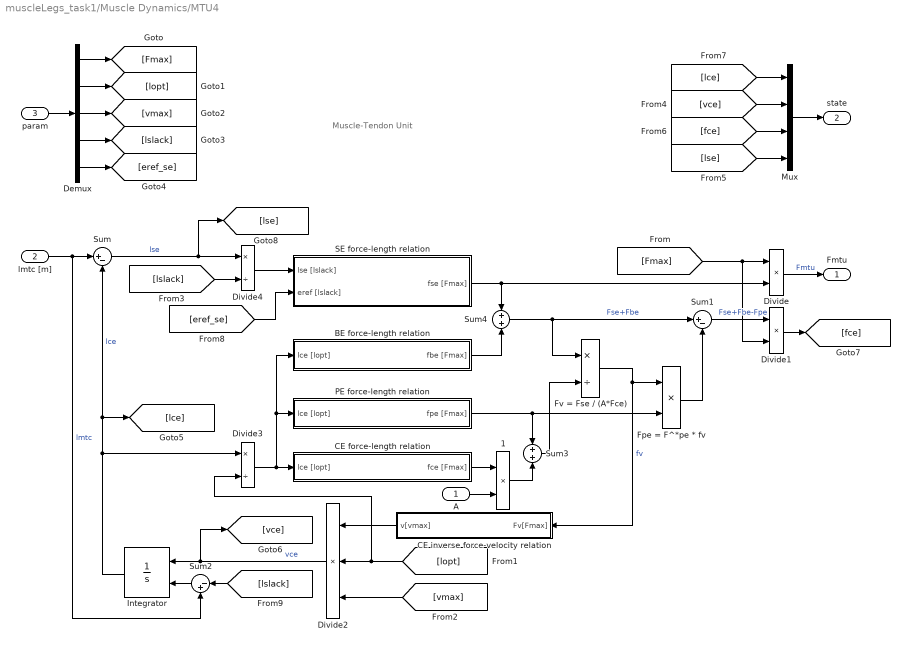
== system muscleLegs_task1/Muscle Dynamics/MTU4 ==
  note: Muscle-Tendon Unit
  A : Inport
  lmtc [m] : Inport  Port=2
  param : Inport  Port=3
  1 : Product  Inputs=**  InputSameDT=on  SaturateOnIntegerOverflow=on  OutDataTypeStr=Inherit: Same as first input
  BE force-length relation : Subsystem
  CE force-length relation : Subsystem
  CE inverse force-velocity relation : Subsystem
  Demux : Demux  Outputs=5
  Divide : Product
  Divide1 : Product
  Divide2 : Product  Inputs=3
  Divide3 : Product  Inputs=*/
  Divide4 : Product  Inputs=*/
  "Fpe = F^*pe * fv " : Product  InputSameDT=on  SaturateOnIntegerOverflow=on  OutDataTypeStr=Inherit: Same as first input
  Fv = Fse / (A*Fce) : Product  Inputs=*/  InputSameDT=on  SaturateOnIntegerOverflow=on  OutDataTypeStr=Inherit: Same as first input
  Integrator : Integrator  InitialConditionSource=external  LowerSaturationLimit=0.05
  Mux : Mux
  PE force-length relation : Subsystem
  SE force-length relation : Subsystem
  Sum : Sum  Inputs=|+-  InputSameDT=on  SaturateOnIntegerOverflow=on  OutDataTypeStr=Inherit: Same as first input
  Sum1 : Sum  Inputs=|+-  InputSameDT=on  SaturateOnIntegerOverflow=on  OutDataTypeStr=Inherit: Same as first input
  Sum2 : Sum  Inputs=|-+  InputSameDT=on  SaturateOnIntegerOverflow=on  OutDataTypeStr=Inherit: Same as first input
  Sum3 : Sum  InputSameDT=on  SaturateOnIntegerOverflow=on  OutDataTypeStr=Inherit: Same as first input
  Sum4 : Sum  InputSameDT=on  SaturateOnIntegerOverflow=on  OutDataTypeStr=Inherit: Same as first input
  Fmtu : Outport  InitialOutput=0  VectorParamsAs1DForOutWhenUnconnected=off
  state : Outport  Port=2  InitialOutput=0  VectorParamsAs1DForOutWhenUnconnected=off
  wires:
  Integrator/1 -> Divide3/1, [lce], Sum/2  "lce"
  Divide3/1 -> CE force-length relation/1(lce [lopt]), PE force-length relation/1(lce [lopt]), BE force-length relation/1(lce [lopt])
  Fv = Fse / (A*Fce)/1 -> CE inverse force-velocity relation/1(Fv[Fmax]), "Fpe = F^*pe * fv "/1  "fv"
  Divide2/1 -> [vce], Integrator/1  "vce"
  lmtc [m]/1 -> Sum/1, Sum2/2  "lmtc"
  Divide/1 -> Fmtu/1  "Fmtu"
  Divide4/1 -> SE force-length relation/1(lse [lslack])
  SE force-length relation/1(fse [Fmax]) -> Sum4/1, Divide/2
  Sum2/1 -> Integrator/2
  [lslack] -> Sum2/1
  CE force-length relation/1(fce [Fmax]) -> 1/1
  PE force-length relation/1(fpe [Fmax]) -> "Fpe = F^*pe * fv "/2, Sum3/1
  1/1 -> Sum3/2
  BE force-length relation/1(fbe [Fmax]) -> Sum4/2
  Sum3/1 -> Fv = Fse / (A*Fce)/2
  CE inverse force-velocity relation/1(v[vmax]) -> Divide2/1
  A/1 -> 1/2
  Sum4/1 -> Sum1/1, Fv = Fse / (A*Fce)/1  "Fse+Fbe"
  "Fpe = F^*pe * fv "/1 -> Sum1/2
  Sum1/1 -> Divide1/1  "Fse+Fbe-Fpe"
  Divide1/1 -> [fce]
  Sum/1 -> [lse], Divide4/1  "lse"
  [lopt] -> Divide2/2, Divide3/2
  [vmax] -> Divide2/3
  [lslack] -> Divide4/2
  param/1 -> Demux/1
  Demux/1 -> [Fmax]
  Demux/2 -> [lopt]
  Demux/4 -> [lslack]
  Demux/3 -> [vmax]
  Demux/5 -> [eref_se]
  [Fmax] -> Divide1/2, Divide/1
  Mux/1 -> state/1
  [lce] -> Mux/1
  [vce] -> Mux/2
  [fce] -> Mux/3
  [lse] -> Mux/4
  [eref_se] -> SE force-length relation/2(eref [lslack])

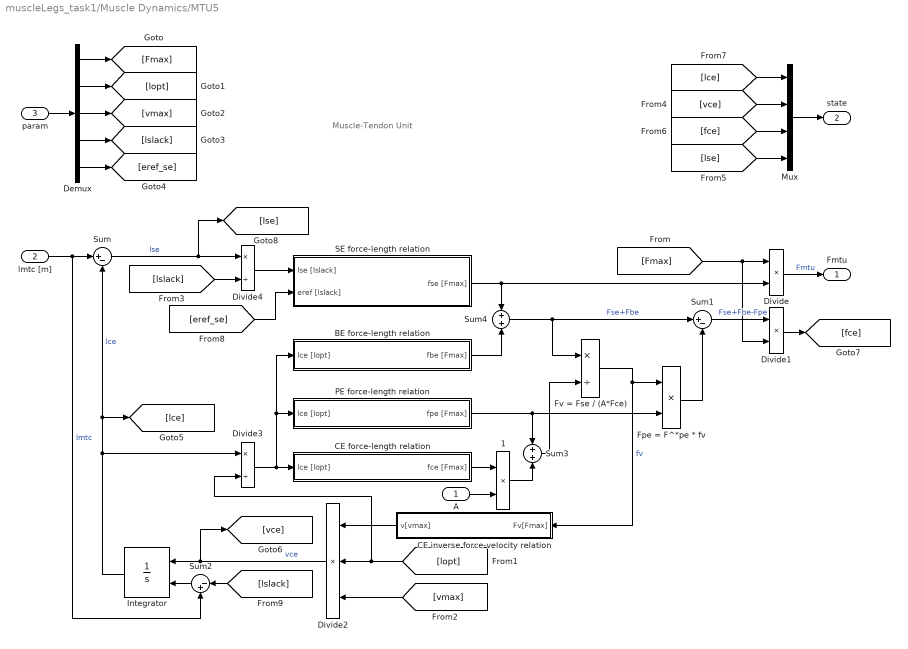
== system muscleLegs_task1/Muscle Dynamics/MTU5 ==
  note: Muscle-Tendon Unit
  A : Inport
  lmtc [m] : Inport  Port=2
  param : Inport  Port=3
  1 : Product  Inputs=**  InputSameDT=on  SaturateOnIntegerOverflow=on  OutDataTypeStr=Inherit: Same as first input
  BE force-length relation : Subsystem
  CE force-length relation : Subsystem
  CE inverse force-velocity relation : Subsystem
  Demux : Demux  Outputs=5
  Divide : Product
  Divide1 : Product
  Divide2 : Product  Inputs=3
  Divide3 : Product  Inputs=*/
  Divide4 : Product  Inputs=*/
  "Fpe = F^*pe * fv " : Product  InputSameDT=on  SaturateOnIntegerOverflow=on  OutDataTypeStr=Inherit: Same as first input
  Fv = Fse / (A*Fce) : Product  Inputs=*/  InputSameDT=on  SaturateOnIntegerOverflow=on  OutDataTypeStr=Inherit: Same as first input
  Integrator : Integrator  InitialConditionSource=external  LowerSaturationLimit=0.05
  Mux : Mux
  PE force-length relation : Subsystem
  SE force-length relation : Subsystem
  Sum : Sum  Inputs=|+-  InputSameDT=on  SaturateOnIntegerOverflow=on  OutDataTypeStr=Inherit: Same as first input
  Sum1 : Sum  Inputs=|+-  InputSameDT=on  SaturateOnIntegerOverflow=on  OutDataTypeStr=Inherit: Same as first input
  Sum2 : Sum  Inputs=|-+  InputSameDT=on  SaturateOnIntegerOverflow=on  OutDataTypeStr=Inherit: Same as first input
  Sum3 : Sum  InputSameDT=on  SaturateOnIntegerOverflow=on  OutDataTypeStr=Inherit: Same as first input
  Sum4 : Sum  InputSameDT=on  SaturateOnIntegerOverflow=on  OutDataTypeStr=Inherit: Same as first input
  Fmtu : Outport  InitialOutput=0  VectorParamsAs1DForOutWhenUnconnected=off
  state : Outport  Port=2  InitialOutput=0  VectorParamsAs1DForOutWhenUnconnected=off
  wires:
  Integrator/1 -> Divide3/1, [lce], Sum/2  "lce"
  Divide3/1 -> CE force-length relation/1(lce [lopt]), PE force-length relation/1(lce [lopt]), BE force-length relation/1(lce [lopt])
  Fv = Fse / (A*Fce)/1 -> CE inverse force-velocity relation/1(Fv[Fmax]), "Fpe = F^*pe * fv "/1  "fv"
  Divide2/1 -> [vce], Integrator/1  "vce"
  lmtc [m]/1 -> Sum/1, Sum2/2  "lmtc"
  Divide/1 -> Fmtu/1  "Fmtu"
  Divide4/1 -> SE force-length relation/1(lse [lslack])
  SE force-length relation/1(fse [Fmax]) -> Sum4/1, Divide/2
  Sum2/1 -> Integrator/2
  [lslack] -> Sum2/1
  CE force-length relation/1(fce [Fmax]) -> 1/1
  PE force-length relation/1(fpe [Fmax]) -> "Fpe = F^*pe * fv "/2, Sum3/1
  1/1 -> Sum3/2
  BE force-length relation/1(fbe [Fmax]) -> Sum4/2
  Sum3/1 -> Fv = Fse / (A*Fce)/2
  CE inverse force-velocity relation/1(v[vmax]) -> Divide2/1
  A/1 -> 1/2
  Sum4/1 -> Sum1/1, Fv = Fse / (A*Fce)/1  "Fse+Fbe"
  "Fpe = F^*pe * fv "/1 -> Sum1/2
  Sum1/1 -> Divide1/1  "Fse+Fbe-Fpe"
  Divide1/1 -> [fce]
  Sum/1 -> [lse], Divide4/1  "lse"
  [lopt] -> Divide2/2, Divide3/2
  [vmax] -> Divide2/3
  [lslack] -> Divide4/2
  param/1 -> Demux/1
  Demux/1 -> [Fmax]
  Demux/2 -> [lopt]
  Demux/4 -> [lslack]
  Demux/3 -> [vmax]
  Demux/5 -> [eref_se]
  [Fmax] -> Divide1/2, Divide/1
  Mux/1 -> state/1
  [lce] -> Mux/1
  [vce] -> Mux/2
  [fce] -> Mux/3
  [lse] -> Mux/4
  [eref_se] -> SE force-length relation/2(eref [lslack])

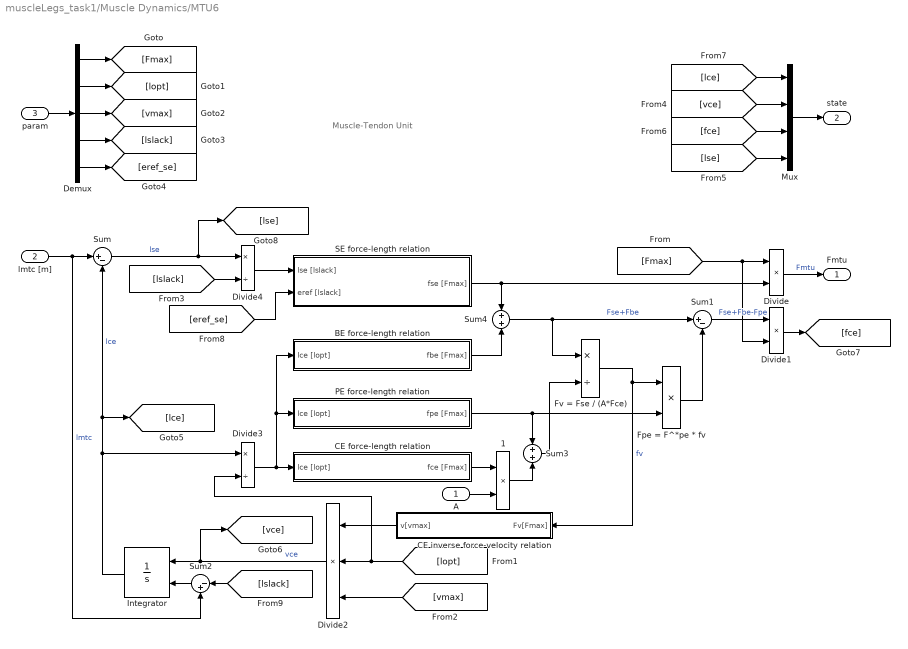
== system muscleLegs_task1/Muscle Dynamics/MTU6 ==
  note: Muscle-Tendon Unit
  A : Inport
  lmtc [m] : Inport  Port=2
  param : Inport  Port=3
  1 : Product  Inputs=**  InputSameDT=on  SaturateOnIntegerOverflow=on  OutDataTypeStr=Inherit: Same as first input
  BE force-length relation : Subsystem
  CE force-length relation : Subsystem
  CE inverse force-velocity relation : Subsystem
  Demux : Demux  Outputs=5
  Divide : Product
  Divide1 : Product
  Divide2 : Product  Inputs=3
  Divide3 : Product  Inputs=*/
  Divide4 : Product  Inputs=*/
  "Fpe = F^*pe * fv " : Product  InputSameDT=on  SaturateOnIntegerOverflow=on  OutDataTypeStr=Inherit: Same as first input
  Fv = Fse / (A*Fce) : Product  Inputs=*/  InputSameDT=on  SaturateOnIntegerOverflow=on  OutDataTypeStr=Inherit: Same as first input
  Integrator : Integrator  InitialConditionSource=external  LowerSaturationLimit=0.05
  Mux : Mux
  PE force-length relation : Subsystem
  SE force-length relation : Subsystem
  Sum : Sum  Inputs=|+-  InputSameDT=on  SaturateOnIntegerOverflow=on  OutDataTypeStr=Inherit: Same as first input
  Sum1 : Sum  Inputs=|+-  InputSameDT=on  SaturateOnIntegerOverflow=on  OutDataTypeStr=Inherit: Same as first input
  Sum2 : Sum  Inputs=|-+  InputSameDT=on  SaturateOnIntegerOverflow=on  OutDataTypeStr=Inherit: Same as first input
  Sum3 : Sum  InputSameDT=on  SaturateOnIntegerOverflow=on  OutDataTypeStr=Inherit: Same as first input
  Sum4 : Sum  InputSameDT=on  SaturateOnIntegerOverflow=on  OutDataTypeStr=Inherit: Same as first input
  Fmtu : Outport  InitialOutput=0  VectorParamsAs1DForOutWhenUnconnected=off
  state : Outport  Port=2  InitialOutput=0  VectorParamsAs1DForOutWhenUnconnected=off
  wires:
  Integrator/1 -> Divide3/1, [lce], Sum/2  "lce"
  Divide3/1 -> CE force-length relation/1(lce [lopt]), PE force-length relation/1(lce [lopt]), BE force-length relation/1(lce [lopt])
  Fv = Fse / (A*Fce)/1 -> CE inverse force-velocity relation/1(Fv[Fmax]), "Fpe = F^*pe * fv "/1  "fv"
  Divide2/1 -> [vce], Integrator/1  "vce"
  lmtc [m]/1 -> Sum/1, Sum2/2  "lmtc"
  Divide/1 -> Fmtu/1  "Fmtu"
  Divide4/1 -> SE force-length relation/1(lse [lslack])
  SE force-length relation/1(fse [Fmax]) -> Sum4/1, Divide/2
  Sum2/1 -> Integrator/2
  [lslack] -> Sum2/1
  CE force-length relation/1(fce [Fmax]) -> 1/1
  PE force-length relation/1(fpe [Fmax]) -> "Fpe = F^*pe * fv "/2, Sum3/1
  1/1 -> Sum3/2
  BE force-length relation/1(fbe [Fmax]) -> Sum4/2
  Sum3/1 -> Fv = Fse / (A*Fce)/2
  CE inverse force-velocity relation/1(v[vmax]) -> Divide2/1
  A/1 -> 1/2
  Sum4/1 -> Sum1/1, Fv = Fse / (A*Fce)/1  "Fse+Fbe"
  "Fpe = F^*pe * fv "/1 -> Sum1/2
  Sum1/1 -> Divide1/1  "Fse+Fbe-Fpe"
  Divide1/1 -> [fce]
  Sum/1 -> [lse], Divide4/1  "lse"
  [lopt] -> Divide2/2, Divide3/2
  [vmax] -> Divide2/3
  [lslack] -> Divide4/2
  param/1 -> Demux/1
  Demux/1 -> [Fmax]
  Demux/2 -> [lopt]
  Demux/4 -> [lslack]
  Demux/3 -> [vmax]
  Demux/5 -> [eref_se]
  [Fmax] -> Divide1/2, Divide/1
  Mux/1 -> state/1
  [lce] -> Mux/1
  [vce] -> Mux/2
  [fce] -> Mux/3
  [lse] -> Mux/4
  [eref_se] -> SE force-length relation/2(eref [lslack])

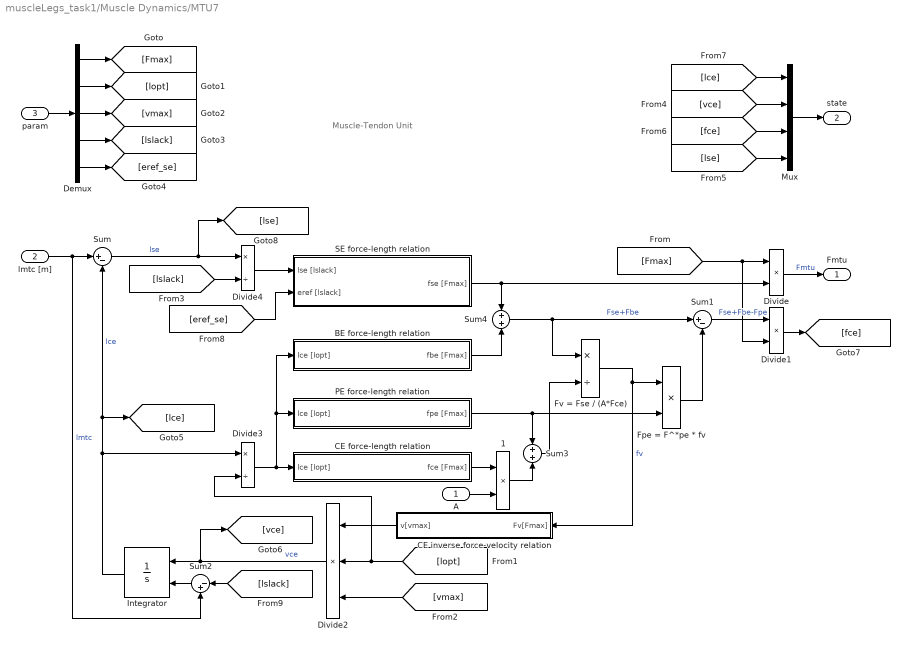
== system muscleLegs_task1/Muscle Dynamics/MTU7 ==
  note: Muscle-Tendon Unit
  A : Inport
  lmtc [m] : Inport  Port=2
  param : Inport  Port=3
  1 : Product  Inputs=**  InputSameDT=on  SaturateOnIntegerOverflow=on  OutDataTypeStr=Inherit: Same as first input
  BE force-length relation : Subsystem
  CE force-length relation : Subsystem
  CE inverse force-velocity relation : Subsystem
  Demux : Demux  Outputs=5
  Divide : Product
  Divide1 : Product
  Divide2 : Product  Inputs=3
  Divide3 : Product  Inputs=*/
  Divide4 : Product  Inputs=*/
  "Fpe = F^*pe * fv " : Product  InputSameDT=on  SaturateOnIntegerOverflow=on  OutDataTypeStr=Inherit: Same as first input
  Fv = Fse / (A*Fce) : Product  Inputs=*/  InputSameDT=on  SaturateOnIntegerOverflow=on  OutDataTypeStr=Inherit: Same as first input
  Integrator : Integrator  InitialConditionSource=external  LowerSaturationLimit=0.05
  Mux : Mux
  PE force-length relation : Subsystem
  SE force-length relation : Subsystem
  Sum : Sum  Inputs=|+-  InputSameDT=on  SaturateOnIntegerOverflow=on  OutDataTypeStr=Inherit: Same as first input
  Sum1 : Sum  Inputs=|+-  InputSameDT=on  SaturateOnIntegerOverflow=on  OutDataTypeStr=Inherit: Same as first input
  Sum2 : Sum  Inputs=|-+  InputSameDT=on  SaturateOnIntegerOverflow=on  OutDataTypeStr=Inherit: Same as first input
  Sum3 : Sum  InputSameDT=on  SaturateOnIntegerOverflow=on  OutDataTypeStr=Inherit: Same as first input
  Sum4 : Sum  InputSameDT=on  SaturateOnIntegerOverflow=on  OutDataTypeStr=Inherit: Same as first input
  Fmtu : Outport  InitialOutput=0  VectorParamsAs1DForOutWhenUnconnected=off
  state : Outport  Port=2  InitialOutput=0  VectorParamsAs1DForOutWhenUnconnected=off
  wires:
  Integrator/1 -> Divide3/1, [lce], Sum/2  "lce"
  Divide3/1 -> CE force-length relation/1(lce [lopt]), PE force-length relation/1(lce [lopt]), BE force-length relation/1(lce [lopt])
  Fv = Fse / (A*Fce)/1 -> CE inverse force-velocity relation/1(Fv[Fmax]), "Fpe = F^*pe * fv "/1  "fv"
  Divide2/1 -> [vce], Integrator/1  "vce"
  lmtc [m]/1 -> Sum/1, Sum2/2  "lmtc"
  Divide/1 -> Fmtu/1  "Fmtu"
  Divide4/1 -> SE force-length relation/1(lse [lslack])
  SE force-length relation/1(fse [Fmax]) -> Sum4/1, Divide/2
  Sum2/1 -> Integrator/2
  [lslack] -> Sum2/1
  CE force-length relation/1(fce [Fmax]) -> 1/1
  PE force-length relation/1(fpe [Fmax]) -> "Fpe = F^*pe * fv "/2, Sum3/1
  1/1 -> Sum3/2
  BE force-length relation/1(fbe [Fmax]) -> Sum4/2
  Sum3/1 -> Fv = Fse / (A*Fce)/2
  CE inverse force-velocity relation/1(v[vmax]) -> Divide2/1
  A/1 -> 1/2
  Sum4/1 -> Sum1/1, Fv = Fse / (A*Fce)/1  "Fse+Fbe"
  "Fpe = F^*pe * fv "/1 -> Sum1/2
  Sum1/1 -> Divide1/1  "Fse+Fbe-Fpe"
  Divide1/1 -> [fce]
  Sum/1 -> [lse], Divide4/1  "lse"
  [lopt] -> Divide2/2, Divide3/2
  [vmax] -> Divide2/3
  [lslack] -> Divide4/2
  param/1 -> Demux/1
  Demux/1 -> [Fmax]
  Demux/2 -> [lopt]
  Demux/4 -> [lslack]
  Demux/3 -> [vmax]
  Demux/5 -> [eref_se]
  [Fmax] -> Divide1/2, Divide/1
  Mux/1 -> state/1
  [lce] -> Mux/1
  [vce] -> Mux/2
  [fce] -> Mux/3
  [lse] -> Mux/4
  [eref_se] -> SE force-length relation/2(eref [lslack])

== system muscleLegs_task1/Neural Control/Stance L ==
  CtrlPar : Inport
  phi_K : Inport  Port=2
  d_phi_K : Inport  Port=3
  Enable : EnablePort
  Constant2 : Constant  Value=0
  Demux : Demux  Outputs=length(vi_Ctrl_st)
  Divide : Product
  Divide1 : Product
  Gain : Gain  Gain=-1
  Gain1 : Gain  Gain=-1
  Sum : Sum  Inputs=|+-
  Sum1 : Sum  Inputs=|+-
  Sum2 : Sum  Inputs=|++
  extension : Saturate  UpperLimit=1  LowerLimit=0.01
  extension1 : Saturate  UpperLimit=1  LowerLimit=0.01
  flexion : Saturate  UpperLimit=1  LowerLimit=0.01
  flexion1 : Saturate  UpperLimit=1  LowerLimit=0.01
  S_VAS : Outport  OutputWhenDisabled=reset  InitialOutput=0
  S_BFSH : Outport  Port=2  OutputWhenDisabled=reset  InitialOutput=0
  S_GLU : Outport  Port=3  OutputWhenDisabled=reset  InitialOutput=0
  S_HFL : Outport  Port=4  OutputWhenDisabled=reset  InitialOutput=0
  wires:
  Divide1/1 -> Sum2/2
  d_phi_K/1 -> Sum1/2
  phi_K/1 -> Sum/2
  Divide/1 -> Sum2/1
  Sum/1 -> Divide/2
  Sum1/1 -> Divide1/2
  Constant2/1 -> Sum1/1
  CtrlPar/1 -> Demux/1
  Demux/1 -> flexion1/1, Gain1/1  "tau_H_st"
  Demux/2 -> Sum/1  "phi_K_tgt_st"
  Demux/3 -> Divide/1  "P_K_st"
  Demux/4 -> Divide1/1  "D_K_st"
  extension/1 -> S_VAS/1
  Gain/1 -> extension/1
  Sum2/1 -> flexion/1, Gain/1
  flexion/1 -> S_BFSH/1
  Gain1/1 -> extension1/1
  extension1/1 -> S_GLU/1
  flexion1/1 -> S_HFL/1

== system muscleLegs_task1/Neural Control/Stance R ==
  CtrlPar : Inport
  phi_K : Inport  Port=2
  d_phi_K : Inport  Port=3
  Enable : EnablePort
  Constant2 : Constant  Value=0
  Demux : Demux  Outputs=length(vi_Ctrl_st)
  Divide : Product
  Divide1 : Product
  Gain : Gain  Gain=-1
  Gain1 : Gain  Gain=-1
  Sum : Sum  Inputs=|+-
  Sum1 : Sum  Inputs=|+-
  Sum2 : Sum  Inputs=|++
  extension : Saturate  UpperLimit=1  LowerLimit=0.01
  extension1 : Saturate  UpperLimit=1  LowerLimit=0.01
  flexion : Saturate  UpperLimit=1  LowerLimit=0.01
  flexion1 : Saturate  UpperLimit=1  LowerLimit=0.01
  S_VAS : Outport  OutputWhenDisabled=reset  InitialOutput=0
  S_BFSH : Outport  Port=2  OutputWhenDisabled=reset  InitialOutput=0
  S_GLU : Outport  Port=3  OutputWhenDisabled=reset  InitialOutput=0
  S_HFL : Outport  Port=4  OutputWhenDisabled=reset  InitialOutput=0
  wires:
  Divide1/1 -> Sum2/2
  d_phi_K/1 -> Sum1/2
  phi_K/1 -> Sum/2
  Divide/1 -> Sum2/1
  Sum/1 -> Divide/2
  Sum1/1 -> Divide1/2
  Constant2/1 -> Sum1/1
  CtrlPar/1 -> Demux/1
  Demux/2 -> Sum/1  "phi_K_tgt_st"
  Demux/3 -> Divide/1  "P_K_st"
  Demux/4 -> Divide1/1  "D_K_st"
  Demux/1 -> flexion1/1, Gain1/1  "tau_H_st"
  Gain1/1 -> extension1/1
  flexion/1 -> S_BFSH/1
  Sum2/1 -> flexion/1, Gain/1
  extension/1 -> S_VAS/1
  Gain/1 -> extension/1
  extension1/1 -> S_GLU/1
  flexion1/1 -> S_HFL/1

== system muscleLegs_task1/Neural Control/Swing L ==
  CtrlPar : Inport
  phi_H : Inport  Port=2
  d_phi_H : Inport  Port=3
  phi_K : Inport  Port=4
  d_phi_K : Inport  Port=5
  Enable : EnablePort
  Constant2 : Constant  Value=0
  Constant3 : Constant  Value=0
  Demux1 : Demux  Outputs=length(vi_Ctrl_sw)
  Divide{,1..3} (4 alike) : Product
  Gain : Gain  Gain=-1
  Gain1 : Gain  Gain=-1
  Gain4 : Gain  Gain=180/pi
  Gain5 : Gain  Gain=180/pi
  Multiport Switch : MultiPortSwitch  DataPortOrder=Zero-based contiguous  Inputs=2  zeroidx=on  SaturateOnIntegerOverflow=off  InputSameDT=off
  Mux4 : Mux  Inputs=2
  Relational Operator : RelationalOperator  Operator=>  OutDataTypeStr=boolean  RndMeth=Simplest  InputSameDT=off
  Scope1 : Scope  NumInputPorts=3
      settings: ActiveDisplayYMinimum=-0.56332  ActiveDisplayYMaximum=0.70659  DataLoggingVariableName=ScopeData2
  Sum{,1,3..4} (4 alike) : Sum  Inputs=|+-
  Sum2 : Sum  Inputs=|++
  Sum5 : Sum  Inputs=|++
  extension : Saturate  UpperLimit=1  LowerLimit=0.01
  extension1 : Saturate  UpperLimit=1  LowerLimit=0.01
  flexion : Saturate  UpperLimit=1  LowerLimit=0.01
  flexion1 : Saturate  UpperLimit=1  LowerLimit=0.01
  phi_L : Fcn  Expr=u(1) - 0.5*u(2)
  S_VAS : Outport  OutputWhenDisabled=reset  InitialOutput=0
  S_BFSH : Outport  Port=2  OutputWhenDisabled=reset  InitialOutput=0
  S_GLU : Outport  Port=3  OutputWhenDisabled=reset  InitialOutput=0
  S_HFL : Outport  Port=4  OutputWhenDisabled=reset  InitialOutput=0
  wires:
  Sum1/1 -> Divide1/2
  Sum/1 -> Divide/2
  Divide1/1 -> Sum2/2
  Constant3/1 -> Sum1/1
  Divide/1 -> Sum2/1
  d_phi_H/1 -> Sum1/2
  Mux4/1 -> phi_L/1
  phi_H/1 -> Mux4/1
  phi_L/1 -> Relational Operator/1, Sum/2, Gain4/1
  Multiport Switch/1 -> Sum3/1, Gain5/1  "phi_K_tgt_sw"
  phi_K/1 -> Sum3/2, Mux4/2
  Divide3/1 -> Sum5/2
  Constant2/1 -> Sum4/1
  Sum4/1 -> Divide3/2
  Divide2/1 -> Sum5/1
  Sum3/1 -> Divide2/2
  d_phi_K/1 -> Sum4/2
  Relational Operator/1 -> Multiport Switch/1, Scope1/2
  Gain4/1 -> Scope1/1
  Gain5/1 -> Scope1/3
  Demux1/1 -> Sum/1  "phi_H_tgt_sw"
  CtrlPar/1 -> Demux1/1
  Demux1/2 -> Divide/1  "P_H_sw"
  Demux1/3 -> Divide1/1  "D_H_sw"
  Demux1/4 -> Multiport Switch/2  "v_phi_K_tgt_sw(1)"
  Demux1/5 -> Multiport Switch/3  "v_phi_K_tgt_sw(2)"
  Demux1/7 -> Divide2/1  "P_K_sw"
  Demux1/8 -> Divide3/1  "D_K_sw"
  Demux1/6 -> Relational Operator/2  "phi_H_ref_sw"
  Sum5/1 -> flexion/1, Gain/1
  Gain/1 -> extension/1
  extension/1 -> S_VAS/1
  flexion/1 -> S_BFSH/1
  Sum2/1 -> Gain1/1, flexion1/1  "tau_H_st"
  Gain1/1 -> extension1/1
  flexion1/1 -> S_HFL/1
  extension1/1 -> S_GLU/1

== system muscleLegs_task1/Neural Control/Swing R ==
  CtrlPar : Inport
  phi_H : Inport  Port=2
  d_phi_H : Inport  Port=3
  phi_K : Inport  Port=4
  d_phi_K : Inport  Port=5
  Enable : EnablePort
  Constant2 : Constant  Value=0
  Constant3 : Constant  Value=0
  Demux1 : Demux  Outputs=length(vi_Ctrl_sw)
  Divide{,1..3} (4 alike) : Product
  Gain : Gain  Gain=-1
  Gain1 : Gain  Gain=-1
  Gain4 : Gain  Gain=180/pi
  Gain5 : Gain  Gain=180/pi
  Multiport Switch : MultiPortSwitch  DataPortOrder=Zero-based contiguous  Inputs=2  zeroidx=on  SaturateOnIntegerOverflow=off  InputSameDT=off
  Mux4 : Mux  Inputs=2
  Relational Operator : RelationalOperator  Operator=>  OutDataTypeStr=boolean  RndMeth=Simplest  InputSameDT=off
  Scope1 : Scope  NumInputPorts=3
      settings: ActiveDisplayYMinimum=-0.56332  ActiveDisplayYMaximum=0.70659  DataLoggingVariableName=ScopeData2
  Sum{,1,3..4} (4 alike) : Sum  Inputs=|+-
  Sum2 : Sum  Inputs=|++
  Sum5 : Sum  Inputs=|++
  extension : Saturate  UpperLimit=1  LowerLimit=0.01
  extension1 : Saturate  UpperLimit=1  LowerLimit=0.01
  flexion : Saturate  UpperLimit=1  LowerLimit=0.01
  flexion1 : Saturate  UpperLimit=1  LowerLimit=0.01
  phi_L : Fcn  Expr=u(1) - 0.5*u(2)
  S_VAS : Outport  OutputWhenDisabled=reset  InitialOutput=0
  S_BFSH : Outport  Port=2  OutputWhenDisabled=reset  InitialOutput=0
  S_GLU : Outport  Port=3  OutputWhenDisabled=reset  InitialOutput=0
  S_HFL : Outport  Port=4  OutputWhenDisabled=reset  InitialOutput=0
  wires:
  Sum1/1 -> Divide1/2
  Sum/1 -> Divide/2
  Divide1/1 -> Sum2/2
  Constant3/1 -> Sum1/1
  Divide/1 -> Sum2/1
  d_phi_H/1 -> Sum1/2
  Mux4/1 -> phi_L/1
  phi_H/1 -> Mux4/1
  phi_L/1 -> Relational Operator/1, Sum/2, Gain4/1
  Multiport Switch/1 -> Sum3/1, Gain5/1  "phi_K_tgt_sw"
  phi_K/1 -> Sum3/2, Mux4/2
  Divide3/1 -> Sum5/2
  Constant2/1 -> Sum4/1
  Sum4/1 -> Divide3/2
  Divide2/1 -> Sum5/1
  Sum3/1 -> Divide2/2
  d_phi_K/1 -> Sum4/2
  Relational Operator/1 -> Multiport Switch/1, Scope1/2
  Gain4/1 -> Scope1/1
  Gain5/1 -> Scope1/3
  Demux1/1 -> Sum/1  "phi_H_tgt_sw"
  CtrlPar/1 -> Demux1/1
  Demux1/2 -> Divide/1  "P_H_sw"
  Demux1/3 -> Divide1/1  "D_H_sw"
  Demux1/4 -> Multiport Switch/2  "v_phi_K_tgt_sw(1)"
  Demux1/5 -> Multiport Switch/3  "v_phi_K_tgt_sw(2)"
  Demux1/7 -> Divide2/1  "P_K_sw"
  Demux1/8 -> Divide3/1  "D_K_sw"
  Demux1/6 -> Relational Operator/2  "phi_H_ref_sw"
  Sum5/1 -> flexion/1, Gain/1
  Gain/1 -> extension/1
  extension/1 -> S_VAS/1
  flexion/1 -> S_BFSH/1
  Sum2/1 -> flexion1/1, Gain1/1  "tau_H_st"
  Gain1/1 -> extension1/1
  extension1/1 -> S_GLU/1
  flexion1/1 -> S_HFL/1
